simulink model "olapfilt"  (Simulink 5.0)
settings: Solver=FixedStepDiscrete  SolverMode=SingleTasking  StartTime=0.0  StopTime=0.05  RelTol=1e-3  AbsTol=1e-6
libraries: dsparch4 x3, dspsrcs4 x1
settings Model: CovMetricSettings=d  Creator=don  LastModifiedBy=mkhan  SaveTime=off  SaveOutput=off  LimitDataPoints=off  IntegerOverflowMsg=none  RTWOptions=-aRollThreshold=2  ExtModeTrigMode=oneshot  ExtModeArmWhenConnect=off  BlockReductionOpt=off  BooleanDataType=off

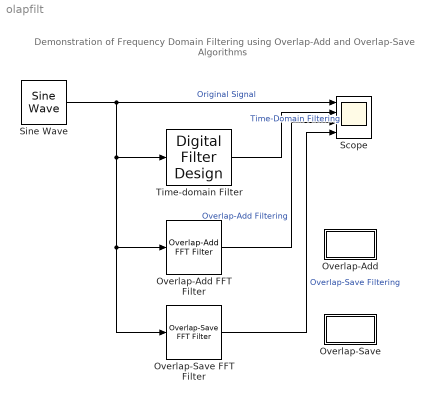
== system olapfilt ==
  note: Demonstration of Frequency Domain Filtering
      | using Overlap-Add and Overlap-Save Algorithms
  Overlap-Add : Subsystem
      settings: RTWFcnNameOpts=Auto  RTWFileNameOpts=Auto
      mask Display: disp('Info')
  Overlap-Add FFT Filter : dsparch4/Overlap-Add FFT Filter  Nfft=64  h=fir1(20,0.2)  output_complexity=Real
  Overlap-Save : Subsystem
      settings: RTWFcnNameOpts=Auto  RTWFileNameOpts=Auto
      mask Display: disp('Info')
  Overlap-Save FFT Filter : dsparch4/Overlap-Save FFT Filter  nfft_in=64  h=fir1(20,0.2)  output_complexity=Real
  Scope : Scope  NumInputPorts=4
      settings: TimeRange=0.05  YMin=-1~-1~-1~-1  YMax=1~1~1~1  SaveToWorkspace=off  SaveName=ScopeData  DataFormat=Array  LimitDataPoints=on  MaxDataPoints=5000
  Sine Wave : dspsrcs4/Sine Wave  Amplitude=1  Frequency=500  Phase=0  SampleMode=Discrete  OutComplex=Real  CompMethod=Trigonometric fcn  TableSize=Speed  SampleTime=1/5000  SamplesPerFrame=1  dType=Double  ResetState=Restart at time zero
  Time-domain Filter : dsparch4/Digital Filter Design
  wires:
  Sine Wave/1 -> Scope/1, Time-domain Filter/1, Overlap-Add FFT Filter/1, Overlap-Save FFT Filter/1  "Original Signal"
  Time-domain Filter/1 -> Scope/2  "Time-Domain Filtering"
  Overlap-Add FFT Filter/1 -> Scope/3  "Overlap-Add Filtering"
  Overlap-Save FFT Filter/1 -> Scope/4  "Overlap-Save Filtering"

== system olapfilt/Overlap-Add ==
  note: Overlap-Add Algorithm
      |
      | This algorithm filters the input signal.  The input is
      | divided into non-overlapping blocks which are linearly
      | convolved with the FIR filter coefficients.
      |
      | The linear convolution of each block is computed
      | by multiplying the DFTs of the block and the filter
      | coefficients, and computing the inverse DFT of the  product.
      |
      | For filter length M and FFT size N, the last M-1 samples
      | of the linear convolution are added to the first M-1
      | samples of the next input sequence.   The first (N-M+1)
      | samples of each summation result are output in sequence.
      |
      | Reference: Proakis and Manolakis, Digital Signal Processing,
      | 3rd ed, Prentice-Hall, Englewood Cliffs, NJ, 1996,
      | pp. 430 - 433.

== system olapfilt/Overlap-Save ==
  note: Overlap Save Algorithm
  note: This algorithm filters the input signal.  The input
      | is divided into overlapping blocks which are circularly
      | convolved with the FIR filter coefficients.
  note: The circular convolution of each block is computed
      | by multiplying the DFTs of the block and the filter
      | coefficients, and computing the inverse DFT of the  product.
  note: For filter length M and FFT size N, the first M-1 points
      | of the circular convolution are invalid and discarded.
      | The remaining (N-M+1) points which are equivalent to
      | the true convolution are "unrolled" as output by the
      | Unbuffer block.
  note: Reference: Oppenheim and Schafer, Discrete-Time Signal
      | Processing, Prentice-Hall, Englewood Cliffs, NJ, 1989,
      | pp. 558 - 560.
